simulink model "can_communcation_test"  (R2023b)
settings: Solver=VariableStepAuto  StartTime=0.0  StopTime=40  RelTol=1e-3
undefined symbols (not defined in the file): canChannel
libraries: canlib x3, canmsglib x2, simulink x1
settings Model: Creator=jcm52  LastModifiedBy=jcm52

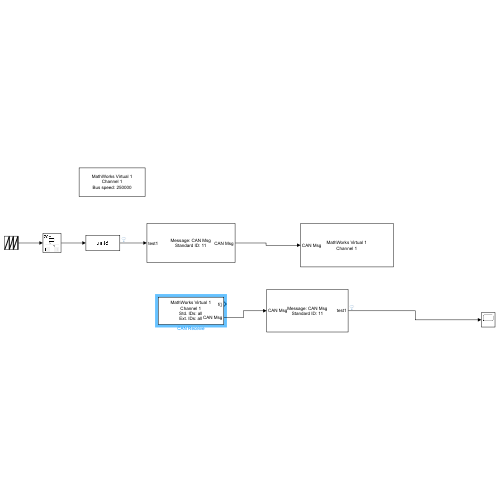
[thumbnail: Simulink's stored preview of the top-level diagram]
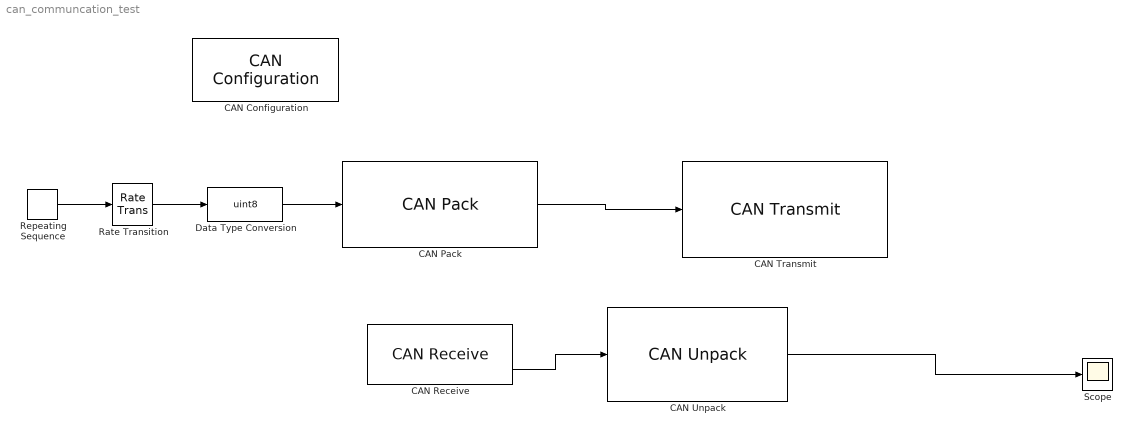
== system can_communcation_test ==
  CAN Configuration : canlib/CAN Configuration  BlockHandle=383.0002  Device=MathWorks Virtual 1 (Channel 1)  DeviceMenu=MathWorks Virtual 1 (Channel 1)  ObjConstructor=canChannel('MathWorks', 'Virtual 1', 1)  BusSpeed=250000  EnableBitParameters=off  AckMode=Normal
  CAN Pack : canmsglib/CAN Pack  MsgList=(none)  MsgName=CAN Msg  MsgIDType=Standard (11-bit identifier)  MsgIdentifier=11  MsgLength=8  Remote=off  ApplyMinMax=off  BusOutput=off  SignalInfo={ 'test1', '0', '8', 'LE', 'unsigned', 'Standard', '0', '1', '0', '-Inf', 'Inf' }
      settings: LibrarySourceBlock=canlib/CAN Pack  DataFormat=manually specified signals
  CAN Receive : canlib/CAN Receive  BlockHandle=384.0002  Device=MathWorks Virtual 1 (Channel 1)  DeviceMenu=MathWorks Virtual 1 (Channel 1)  ObjConstructor=canChannel('MathWorks', 'Virtual 1', 1)  EnableStandardIDsFilter=off  StdIDsCombo=Allow all  StandardIDs=0  EnableExtendedIDsFilter=off  ExtIDsCombo=Allow all  ExtendedIDs=0  SampleTime=0.005  MsgsPerTimestep=all  InternalFilterUpdateStatus=on  BusOutput=off
  CAN Transmit : canlib/CAN Transmit  BlockHandle=385.0002  Device=MathWorks Virtual 1 (Channel 1)  DeviceMenu=MathWorks Virtual 1 (Channel 1)  ObjConstructor=canChannel('MathWorks', 'Virtual 1', 1)  EnableEventTransmit=off  EnablePeriodicTransmit=off  MessagePeriod=0.005
  CAN Unpack : canmsglib/CAN Unpack  MsgList=(none)  MsgName=CAN Msg  MsgIDType=Standard (11-bit identifier)  MsgIdentifier=11  MsgLength=8  SignalInfo={ 'test1', '0', '8', 'LE', 'unsigned', 'Standard', '0', '1', '0', '-Inf', 'Inf' }  IDPort=off  TimestampPort=off  ErrorPort=off  RemotePort=off  LengthPort=off  StatusPort=off  ApplyMinMax=off
      settings: LibrarySourceBlock=canlib/CAN Unpack
  Data Type Conversion : DataTypeConversion  OutDataTypeStr=uint8  SaturateOnIntegerOverflow=off  RndMeth=Floor
  Rate Transition : RateTransition  OutPortSampleTime=0.0001
  Repeating Sequence : simulink/Sources/Repeating Sequence  rep_seq_t=[0 2 4]  rep_seq_y=[0 2 4]
  Scope : Scope
  wires:
  CAN Pack/1 -> CAN Transmit/1
  CAN Receive/2 -> CAN Unpack/1
  CAN Unpack/1 -> Scope/1
  Data Type Conversion/1 -> CAN Pack/1
  Repeating Sequence/1 -> Rate Transition/1
  Rate Transition/1 -> Data Type Conversion/1
